simulink model "sequence"  (R2024b)
settings: Solver=FixedStepDiscrete  StartTime=0.0  StopTime=10.0  FixedStep=0.1  RelTol=1e-3  EnableMultiTasking=on
libraries: stm32f4xxblockslib x3, stm32blockslib x2
settings Model: STM32="{\"DigitalPortWrite\":[{\"ID\":\"untitled:2\"},{\"ID\":\"untitled:3\"},{\"ID\":\"untitled:4\"},{\"ID\":\"sequence:4\"},{\"ID\":\"sequence:3\"},{\"ID\":\"sequence:2\"}],\"UARTRead\":[{\"ID\":\"untitled:5\"},{\"ID\":\"sequence:5\"}],\"UARTWrite\":[{\"ID\":\"untitled:6\"},{\"ID\":\"sequence:6\"}]}"  Creator=mivia  LastModifiedBy=mivia
settings OptimizationCC: DefaultParameterBehavior=Inlined  EnhancedBackFolding=on  PassReuseOutputArgsAs=Individual arguments  ZeroExternalMemoryAtStartup=off  ZeroInternalMemoryAtStartup=off  MaxStackSize=512  OptimizeBlockOrder=speed  DifferentSizesBufferReuse=on  OptimizationCustomize=off  EfficientTunableParamExpr=on
settings DebuggingCC: ParameterTunabilityLossMsg=error
settings HardwareCC: ProdBitPerPointer=32  ProdBitPerSizeT=32  ProdBitPerPtrDiffT=32  ProdLargestAtomicInteger=Long  ProdLargestAtomicFloat=Double  ProdWordSize=32  ProdLongLongMode=on  ProdHWDeviceType=ARM Compatible->ARM Cortex-M
settings RTWCC: Description=Embedded Coder  SystemTargetFile=ert.tlc  HardwareBoard=STM32G4xx Based  TemplateMakefile=ert_default_tmf  Toolchain=GNU Tools for ARM Embedded Processors
settings CodeAppCC: ForceParamTrailComments=on  IgnoreCustomStorageClasses=off  OperatorAnnotations=on  SimulinkDataObjDesc=on  SFDataObjDesc=on  InsertBlockDesc=on
settings ERTTargetCC: TargetLangStandard=C99 (ISO)  CodeReplacementLibrary=ARM Cortex-M  SupportVariableSizeSignals=on  ExtModeTransport=3  ExtModeStaticAlloc=on  ExtModeStaticAllocSize=2048  ExtModeMexFile=ext_xcp  ExtModeIntrfLevel=Level2 - Open

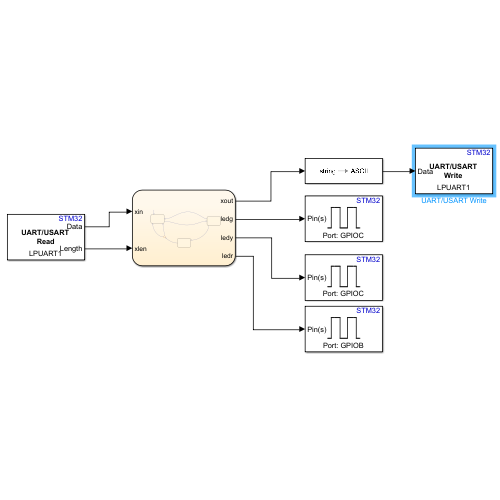
[thumbnail: Simulink's stored preview of the top-level diagram]
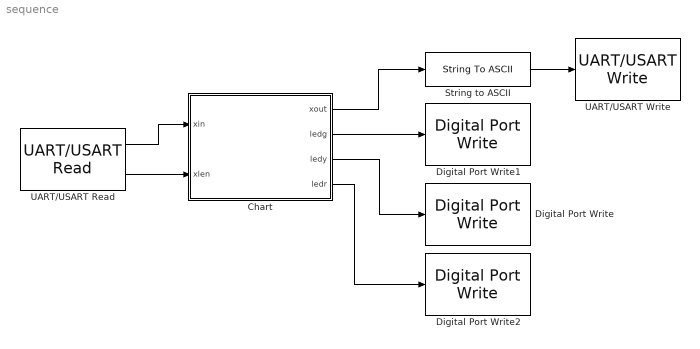
== system sequence ==
  Chart : Stateflow chart  TreatAsAtomicUnit=on
  Digital Port Write : stm32f4xxblockslib/Digital Port Write  PortName=GPIOC  PinNumber=[12]  ReadOperation=off  IOAsArray=on  EnableSimPort=off  hoistedMaskSrc=ECSoC/ECSimCodegen/Digital Port Write
      settings: LibrarySourceBlock=stm32g4xxblockslib/Digital Port Write
  Digital Port Write1 : stm32f4xxblockslib/Digital Port Write  PortName=GPIOC  PinNumber=[10]  ReadOperation=off  IOAsArray=on  EnableSimPort=off  hoistedMaskSrc=ECSoC/ECSimCodegen/Digital Port Write
      settings: LibrarySourceBlock=stm32g4xxblockslib/Digital Port Write
  Digital Port Write2 : stm32f4xxblockslib/Digital Port Write  PortName=GPIOB  PinNumber=[8]  ReadOperation=off  IOAsArray=on  EnableSimPort=off  hoistedMaskSrc=ECSoC/ECSimCodegen/Digital Port Write
      settings: LibrarySourceBlock=stm32g4xxblockslib/Digital Port Write
  String to ASCII : StringToASCII  OutputVectorSize=3
  UART/USART Read : stm32blockslib/UART//USART Read  UARTModule=LPUART1  DataType=uint8  DataLength=1  BlockingMode=off  BlockingTimeout=0.1  OutputLength=on  OutputStatus=off  SampleTime=-1
      settings: LibrarySourceBlock=stm32g4xxblockslib/UART//USART Read
  UART/USART Write : stm32blockslib/UART//USART Write  UARTModule=LPUART1  LengthOfDataToSend=off  BlockingMode=off  BlockingTimeout=0.1  OutputStatus=off
      settings: LibrarySourceBlock=stm32g4xxblockslib/UART//USART Write
  wires:
  Chart/2(ledg) -> Digital Port Write1/1
  Chart/3(ledy) -> Digital Port Write/1
  Chart/4(ledr) -> Digital Port Write2/1
  UART/USART Read/1 -> Chart/1(xin)
  Chart/1(xout) -> String to ASCII/1
  String to ASCII/1 -> UART/USART Write/1
  UART/USART Read/2 -> Chart/2(xlen)

== stateflow chart sequence/Chart ==
  state waiting_a
    en: ledg = ON;
    ex: ledg = OFF;
  state waiting_b
    en: ledy = ON;
    ex: ledy = OFF;
  state out
    en: xout="eos";
    ex: xout="";
  state waiting_c
    en: ledr = ON;
    ex: ledr = OFF;
  (default) -> waiting_a
  waiting_b -> waiting_a [order 1] : [xlen >0 && xin ~= 'b' && xin ~= 'a']
  waiting_a -> waiting_b : [xlen >0 && xin == 'a']
  out -> waiting_a
  (junction 9) -> waiting_a [order 1] : [xin ~= 'c']
  waiting_b -> waiting_c [order 2] : [xlen >0 && xin == 'b']
  (junction 9) -> out [order 2] : [xin == 'c']
  waiting_c -> (junction 9) : [xlen > 0]
  data: xin input uint8; xout output string; OFF constant double =0; ON constant double =1; ledg output; ledy output; ledr output; xlen input
